simulink model "exercise"  (R2024b)
settings: Solver=VariableStepAuto  StartTime=0.0  StopTime=10.0  RelTol=1e-3
settings Model: Creator=Nergigante  LastModifiedBy=Nergigante

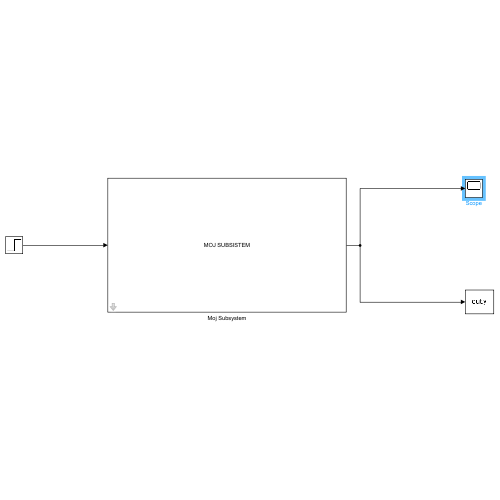
[thumbnail: Simulink's stored preview of the top-level diagram]
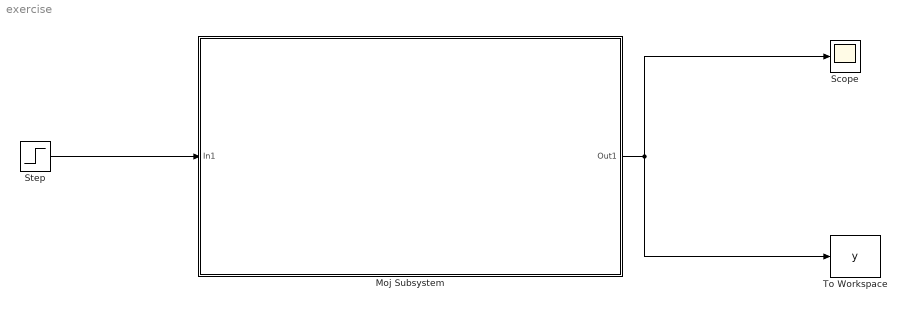
== system exercise ==
  Moj Subsystem : Subsystem  mask{a_0=2, a_1=3, y_0=0, dy_0=1}
      mask Display: disp('MOJ SUBSISTEM');
  Scope : Scope
  Step : Step  SampleTime=0
  To Workspace : ToWorkspace  VariableName=y  SampleTime=-1
      settings: Save2DSignal=2-D array (concatenate along first dimension)
  wires:
  Moj Subsystem/1(Out1) -> To Workspace/1, Scope/1
  Step/1 -> Moj Subsystem/1(In1)

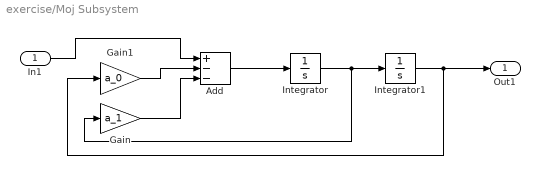
== system exercise/Moj Subsystem ==
  In1 : Inport
  Add : Sum  Inputs=+--
  Gain : Gain  Gain=a_1
  Gain1 : Gain  Gain=a_0
  Integrator : Integrator  InitialCondition=dy_0
  Integrator1 : Integrator  InitialCondition=y_0
  Out1 : Outport
  wires:
  Gain1/1 -> Add/2
  In1/1 -> Add/1
  Integrator1/1 -> Out1/1, Gain1/1
  Gain/1 -> Add/3
  Add/1 -> Integrator/1
  Integrator/1 -> Gain/1, Integrator1/1
